simulink model "example3"  (R2013b)
settings: Solver=ode45  StartTime=0.0  StopTime=20  FixedStep=0.01  RelTol=1e-3
settings Model: PauseTimes=18  Creator=Jin  LastModifiedBy=Jin

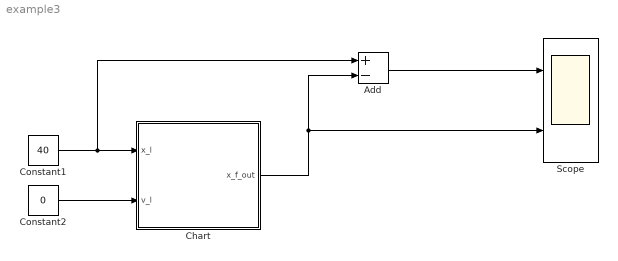
== system example3 ==
  Add : Sum  Inputs=+-
  Chart : Stateflow chart  TreatAsAtomicUnit=on
  Constant1 : Constant  Value=40
  Constant2 : Constant  Value=0
  Scope : Scope  NumInputPorts=2
      settings: YMin=-5~-5  YMax=5~5
  wires:
  Add/1 -> Scope/1
  Constant1/1 -> Add/1, Chart/1(x_l)
  Constant2/1 -> Chart/2(v_l)
  Chart/1(x_f_out) -> Add/2, Scope/2

== stateflow chart example3/Chart ==
  settings: updateMethod=CONTINUOUS
  state Drive
    du:
    x_f_dot = pow(x_l - x_f - 1, 0.5);
    x_f_out = x_f;
  state Collision
    du:
    x_f_dot = 0;
    x_f_out = x_f;
  (default) -> Drive : {x_f = 0;}
  Drive -> Collision : [pow(x_l - x_f - 2, 0.5) <= 0]
  data: x_f local double; x_f_out output double; x_l input double; v_l input
  data x_f settings: updateMethod=SF_CONTINUOUS_TIME_DATA
